simulink model "s1"  (R2022a)
settings: Solver=VariableStepAuto  StartTime=0.0  StopTime=10.0  RelTol=1e-3
settings Model: Creator=PC  LastModifiedBy=PC

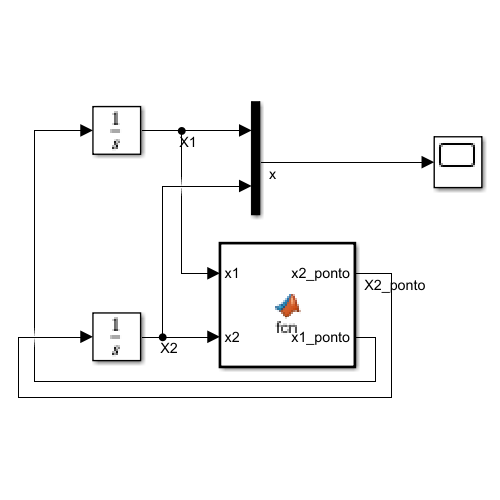
[thumbnail: Simulink's stored preview of the top-level diagram]
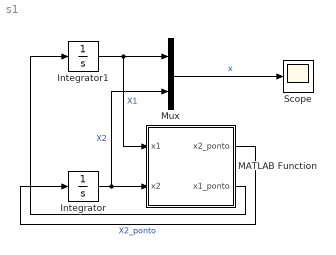
== system s1 ==
  Integrator : Integrator
  Integrator1 : Integrator
  MATLAB Function : MATLAB Function  TreatAsAtomicUnit=on
  Mux : Mux  Inputs=2
  Scope : Scope
  wires:
  MATLAB Function/1(x2_ponto) -> Integrator/1  "X2_ponto"
  MATLAB Function/2(x1_ponto) -> Integrator1/1
  Integrator/1 -> MATLAB Function/2(x2), Mux/2  "X2"
  Mux/1 -> Scope/1  "x"
  Integrator1/1 -> Mux/1, MATLAB Function/1(x1)  "X1"

== matlab function s1/MATLAB Function ==
  data: x1 input; x2_ponto output; x2 input; x1_ponto output
function [x2_ponto,x1_ponto]= fcn(x1,x2)

mi=0.1;
x1_ponto=mi - x1^2;
x2_ponto= -x2;
